simulink model "kinSwCtrl_v2"  (R2015a)
settings: Solver=ode45  StartTime=0.0  StopTime=t_sim  RelTol=1e-3
InitFcn:
  | set_kinSwCtrl_v2;
StopFcn:
  | plot_kinSwCtrl2;
values from neighbouring files (symbols this model uses):
  alpha_0 = 120*pi/180    (= 2.09439510239)    [set_kinSwCtrl_v2.m]    (also in set_kinSwCtrl_v2_2.m)
  alpha_min = 90*pi/180    (= 1.57079632679)    [set_kinSwCtrl_v2.m]    (also in set_kinSwCtrl_v2_2.m = 1.3962634016)
  l_min = 0.7    [set_kinSwCtrl_v2.m]    (also in set_kinSwCtrl_v2_2.m)
  v_alpha = (alpha_min-alpha_0)/t_sim    (= -0.523598775598)    [set_kinSwCtrl_v2.m]    (also in set_kinSwCtrl_v2_2.m = -0.436332312999)
libraries: simulink x1
settings Model: Creator=smsong  LastModifiedBy=smsong

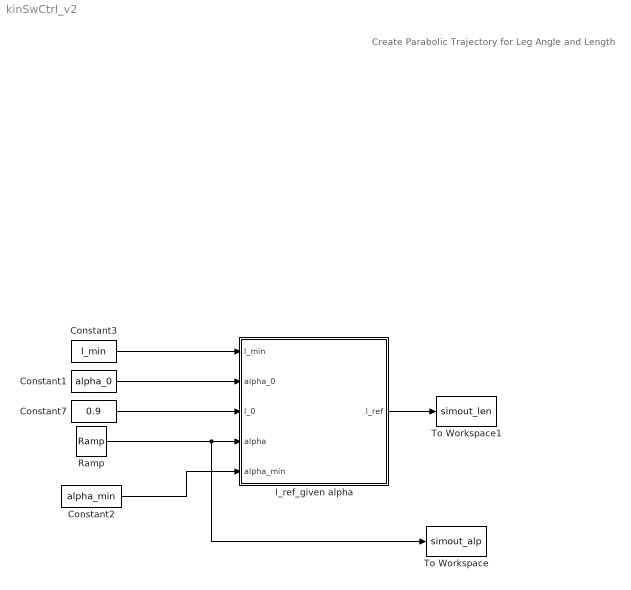
== system kinSwCtrl_v2 ==
  note: Create Parabolic
      | Trajectory for Leg Angle and Length
  Constant1 : Constant  Value=alpha_0
  Constant2 : Constant  Value=alpha_min
  Constant3 : Constant  Value=l_min
  Constant7 : Constant  Value=0.9
  Ramp : simulink/Sources/Ramp  slope=v_alpha  start=0  X0=alpha_0
  To Workspace : ToWorkspace  VariableName=simout_alp  SaveFormat=Structure With Time  SampleTime=-1
  To Workspace1 : ToWorkspace  VariableName=simout_len  SaveFormat=Structure With Time  SampleTime=-1
  l_ref_given alpha : Subsystem
  wires:
  Ramp/1 -> To Workspace/1, l_ref_given alpha/4(alpha)
  Constant7/1 -> l_ref_given alpha/3(l_0)
  Constant1/1 -> l_ref_given alpha/2(alpha_0)
  Constant2/1 -> l_ref_given alpha/5(alpha_min)
  Constant3/1 -> l_ref_given alpha/1(l_min)
  l_ref_given alpha/1(l_ref) -> To Workspace1/1

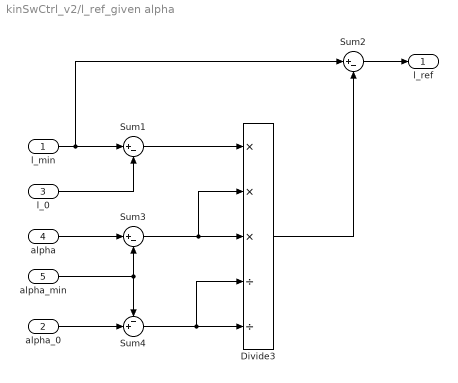
== system kinSwCtrl_v2/l_ref_given alpha ==
  l_min : Inport
  alpha_0 : Inport  Port=2
  l_0 : Inport  Port=3
  alpha : Inport  Port=4
  alpha_min : Inport  Port=5
  Divide3 : Product  Inputs=***//
  Sum1 : Sum  Inputs=|+-
  Sum2 : Sum  Inputs=|+-
  Sum3 : Sum  Inputs=|+-
  Sum4 : Sum  Inputs=-+|
  l_ref : Outport
  wires:
  l_min/1 -> Sum2/1, Sum1/1
  l_0/1 -> Sum1/2
  Sum2/1 -> l_ref/1
  Sum1/1 -> Divide3/1
  alpha/1 -> Sum3/1
  alpha_min/1 -> Sum4/1, Sum3/2
  Sum3/1 -> Divide3/2, Divide3/3
  alpha_0/1 -> Sum4/2
  Sum4/1 -> Divide3/4, Divide3/5
  Divide3/1 -> Sum2/2
